simulink model "simulation_impulse"  (R2023b)
settings: Solver=VariableStepAuto  StartTime=0  StopTime=t_end  RelTol=1e-3
InitFcn:
  | param = plant_param();
undefined symbols (not defined in the file or in its folder): ue, xe
settings Model: Creator=block  LastModifiedBy=MPC5
settings DataIOCC: SaveFormat=StructureWithTime
settings OptimizationCC: BlockReduction=off  BufferReuse=off
settings DebuggingCC: AlgebraicLoopMsg=none

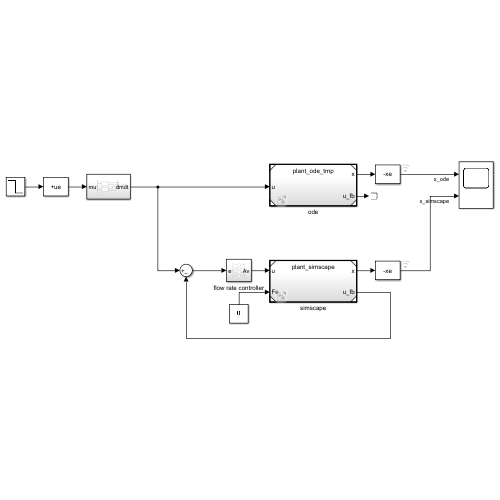
[thumbnail: Simulink's stored preview of the top-level diagram]
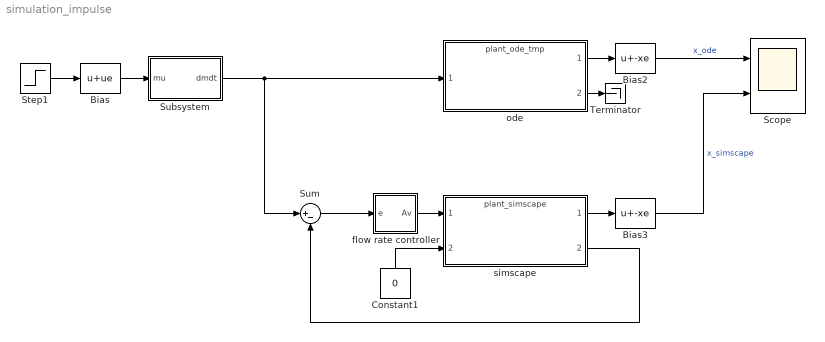
== system simulation_impulse ==
  Bias : Bias  Bias=ue  SaturateOnIntegerOverflow=off
  Bias2 : Bias  Bias=-xe  SaturateOnIntegerOverflow=off
  Bias3 : Bias  Bias=-xe  SaturateOnIntegerOverflow=off
  Constant1 : Constant  Value=0
  Scope : Scope  NumInputPorts=2
  Step1 : Step  Time=0.01  Before=100  After=0  SampleTime=0
  Subsystem : Subsystem
  Sum : Sum  Inputs=|+-
  Terminator : Terminator
  flow rate controller : Subsystem
  ode : ModelReference  ModelNameDialog=plant_ode_tmp  SimulationMode=Normal  ModelReferenceVersion=1.31
  simscape : ModelReference  ModelNameDialog=plant_simscape  SimulationMode=Normal  ModelReferenceVersion=1.82
  wires:
  Bias2/1 -> Scope/1  "x_ode"
  simscape/1 -> Bias3/1
  ode/1 -> Bias2/1
  Bias3/1 -> Scope/2  "x_simscape"
  ode/2 -> Terminator/1
  Step1/1 -> Bias/1
  Bias/1 -> Subsystem/1(mu)
  Subsystem/1(dmdt) -> ode/1, Sum/1
  Sum/1 -> flow rate controller/1(e)
  Constant1/1 -> simscape/2
  flow rate controller/1(Av) -> simscape/1
  simscape/2 -> Sum/2

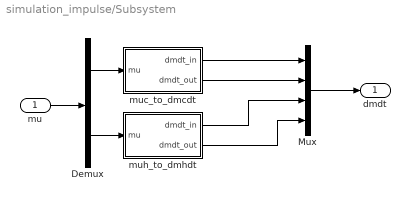
== system simulation_impulse/Subsystem ==
  mu : Inport
  Demux : Demux  Outputs=2
  Mux : Mux
  muc_to_dmcdt : Subsystem
  muh_to_dmhdt : Subsystem
  dmdt : Outport
  wires:
  Demux/1 -> muc_to_dmcdt/1(mu)
  muc_to_dmcdt/1(dmdt_in) -> Mux/1
  muc_to_dmcdt/2(dmdt_out) -> Mux/2
  Demux/2 -> muh_to_dmhdt/1(mu)
  muh_to_dmhdt/1(dmdt_in) -> Mux/3
  muh_to_dmhdt/2(dmdt_out) -> Mux/4
  mu/1 -> Demux/1
  Mux/1 -> dmdt/1

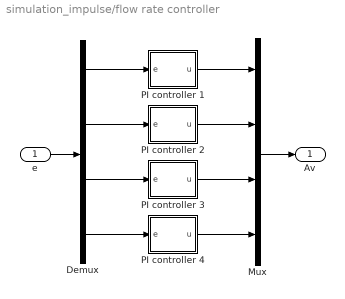
== system simulation_impulse/flow rate controller ==
  e : Inport
  Demux : Demux
  Mux : Mux
  PI controller 1 : Subsystem
  PI controller 2 : Subsystem
  PI controller 3 : Subsystem
  PI controller 4 : Subsystem
  Av : Outport
  wires:
  e/1 -> Demux/1
  Mux/1 -> Av/1
  Demux/2 -> PI controller 2/1(e)
  PI controller 2/1(u) -> Mux/2
  Demux/1 -> PI controller 1/1(e)
  PI controller 1/1(u) -> Mux/1
  PI controller 3/1(u) -> Mux/3
  PI controller 4/1(u) -> Mux/4
  Demux/3 -> PI controller 3/1(e)
  Demux/4 -> PI controller 4/1(e)

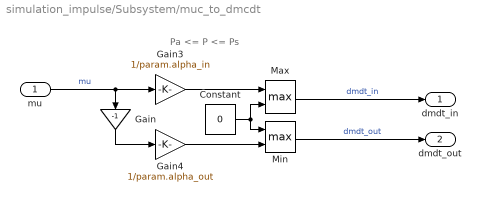
== system simulation_impulse/Subsystem/muc_to_dmcdt ==
  note: Pa <= P <= Ps
  mu : Inport
  Constant : Constant  Value=0
  Gain : Gain  Gain=-1
  Gain3 : Gain  Gain=1/param.alpha_in
  Gain4 : Gain  Gain=1/param.alpha_out
  Max : MinMax  Function=max  Inputs=2
  Min : MinMax  Function=max  Inputs=2
  dmdt_in : Outport
  dmdt_out : Outport  Port=2
  wires:
  Gain3/1 -> Max/1
  Constant/1 -> Max/2, Min/1
  Gain/1 -> Gain4/1
  mu/1 -> Gain3/1, Gain/1  "mu"
  Gain4/1 -> Min/2
  Min/1 -> dmdt_out/1  "dmdt_out"
  Max/1 -> dmdt_in/1  "dmdt_in"

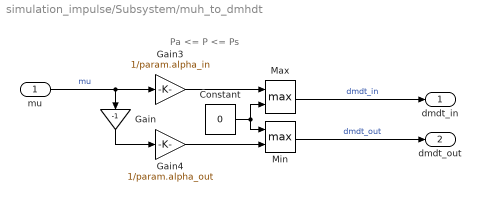
== system simulation_impulse/Subsystem/muh_to_dmhdt ==
  note: Pa <= P <= Ps
  mu : Inport
  Constant : Constant  Value=0
  Gain : Gain  Gain=-1
  Gain3 : Gain  Gain=1/param.alpha_in
  Gain4 : Gain  Gain=1/param.alpha_out
  Max : MinMax  Function=max  Inputs=2
  Min : MinMax  Function=max  Inputs=2
  dmdt_in : Outport
  dmdt_out : Outport  Port=2
  wires:
  Gain3/1 -> Max/1
  Constant/1 -> Max/2, Min/1
  Gain/1 -> Gain4/1
  mu/1 -> Gain3/1, Gain/1  "mu"
  Gain4/1 -> Min/2
  Min/1 -> dmdt_out/1  "dmdt_out"
  Max/1 -> dmdt_in/1  "dmdt_in"

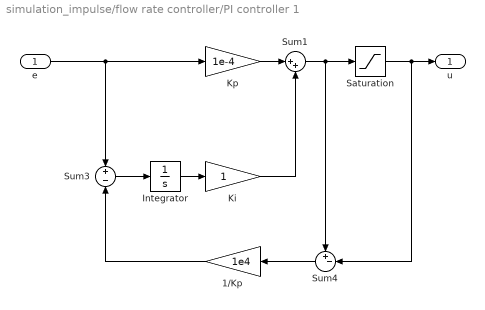
== system simulation_impulse/flow rate controller/PI controller 1 ==
  e : Inport
  1/Kp : Gain  Gain=1e4
  Integrator : Integrator
  Ki : Gain
  Kp : Gain  Gain=1e-4
  Saturation : Saturate  UpperLimit=param.Av  LowerLimit=0
  Sum1 : Sum  Inputs=|++
  Sum3 : Sum  Inputs=+|-
  Sum4 : Sum  Inputs=+-|
  u : Outport
  wires:
  Sum4/1 -> 1/Kp/1
  1/Kp/1 -> Sum3/2
  Sum3/1 -> Integrator/1
  Saturation/1 -> u/1, Sum4/2
  Ki/1 -> Sum1/2
  Kp/1 -> Sum1/1
  Sum1/1 -> Saturation/1, Sum4/1
  e/1 -> Kp/1, Sum3/1
  Integrator/1 -> Ki/1

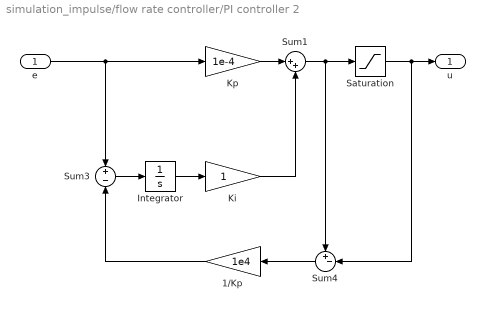
== system simulation_impulse/flow rate controller/PI controller 2 ==
  e : Inport
  1/Kp : Gain  Gain=1e4
  Integrator : Integrator
  Ki : Gain
  Kp : Gain  Gain=1e-4
  Saturation : Saturate  UpperLimit=param.Av  LowerLimit=0
  Sum1 : Sum  Inputs=|++
  Sum3 : Sum  Inputs=+|-
  Sum4 : Sum  Inputs=+-|
  u : Outport
  wires:
  Integrator/1 -> Ki/1
  e/1 -> Sum3/1, Kp/1
  Sum1/1 -> Sum4/1, Saturation/1
  Kp/1 -> Sum1/1
  Ki/1 -> Sum1/2
  Saturation/1 -> Sum4/2, u/1
  Sum3/1 -> Integrator/1
  1/Kp/1 -> Sum3/2
  Sum4/1 -> 1/Kp/1

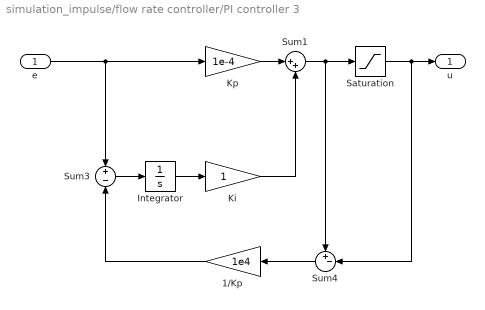
== system simulation_impulse/flow rate controller/PI controller 3 ==
  e : Inport
  1/Kp : Gain  Gain=1e4
  Integrator : Integrator
  Ki : Gain
  Kp : Gain  Gain=1e-4
  Saturation : Saturate  UpperLimit=param.Av  LowerLimit=0
  Sum1 : Sum  Inputs=|++
  Sum3 : Sum  Inputs=+|-
  Sum4 : Sum  Inputs=+-|
  u : Outport
  wires:
  Integrator/1 -> Ki/1
  e/1 -> Sum3/1, Kp/1
  Sum1/1 -> Sum4/1, Saturation/1
  Kp/1 -> Sum1/1
  Ki/1 -> Sum1/2
  Saturation/1 -> Sum4/2, u/1
  Sum3/1 -> Integrator/1
  1/Kp/1 -> Sum3/2
  Sum4/1 -> 1/Kp/1

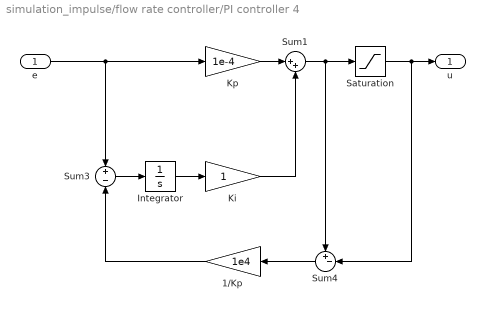
== system simulation_impulse/flow rate controller/PI controller 4 ==
  e : Inport
  1/Kp : Gain  Gain=1e4
  Integrator : Integrator
  Ki : Gain
  Kp : Gain  Gain=1e-4
  Saturation : Saturate  UpperLimit=param.Av  LowerLimit=0
  Sum1 : Sum  Inputs=|++
  Sum3 : Sum  Inputs=+|-
  Sum4 : Sum  Inputs=+-|
  u : Outport
  wires:
  Integrator/1 -> Ki/1
  e/1 -> Sum3/1, Kp/1
  Sum1/1 -> Sum4/1, Saturation/1
  Kp/1 -> Sum1/1
  Ki/1 -> Sum1/2
  Saturation/1 -> Sum4/2, u/1
  Sum3/1 -> Integrator/1
  1/Kp/1 -> Sum3/2
  Sum4/1 -> 1/Kp/1
